simulink model "SimControladorPI"  (R2025b)
settings: Solver=VariableStepAuto  StartTime=0.0  StopTime=tfin  MaxStep=0.01  RelTol=1e-3
values from neighbouring files (symbols this model uses):
  A = max(U)    [AllModels.m]    (also in ConfigurarControl.m = 40; Danier.m; Prueba2.m = 40; PruebaSegundoorden.m)
  den = [tao 1]    [ConfigurarControl.m]    (also in Prueba2.m)
  Kc = 2.5    [ConfigurarControl.m]    (also in Prueba2.m)
  Kc_d = 0.5    [ConfigurarControl.m]    (also in Prueba2.m = 0.2)
  Kc_i = 0.5    [ConfigurarControl.m]    (also in Prueba2.m)
  num = Kp    (= 0.83)    [ConfigurarControl.m]    (also in Prueba2.m)
  t_d = ti_d*0.2    (= 3)    [Prueba2.m]
  tdead = 27.8    [ConfigurarControl.m]    (also in Prueba2.m)
  tesc = 5    [ConfigurarControl.m]    (also in Prueba2.m)
  ti = 10    [ConfigurarControl.m]    (also in Prueba2.m = 20)
libraries: slpidlib x1
settings Model: Creator=b03s217  LastModifiedBy=JF
settings SolverCC: AlgebraicLoopSolver=TrustRegion
settings DebuggingCC: UnconnectedInputMsg=warning  UnconnectedOutputMsg=warning  UnconnectedLineMsg=warning
settings ModelReferenceCC: EnableRefExpFcnMdlSchedulingChecks=on
settings RTWCC: GPUComputeCapability=3.5  DLArmComputeVersion=19.05

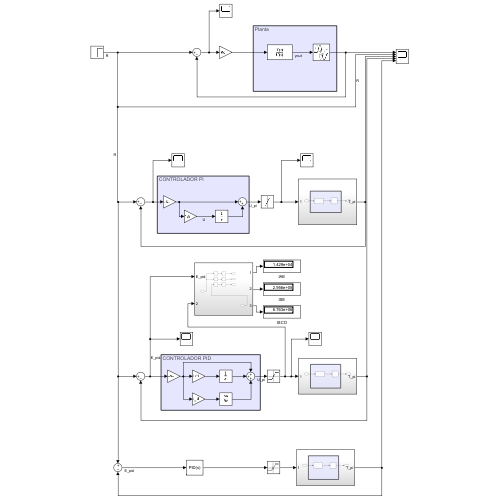
[thumbnail: Simulink's stored preview of the top-level diagram]
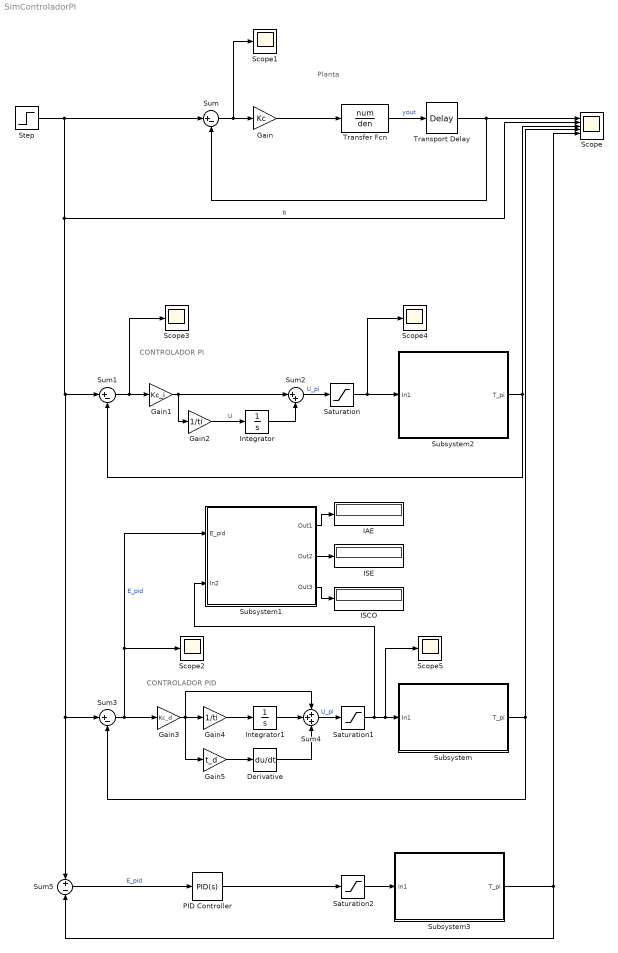
== system SimControladorPI ==
  note: CONTROLADOR PI
  note: CONTROLADOR PID
  note: Planta
  Derivative : Derivative
  Gain : Gain  Gain=Kc
  Gain1 : Gain  Gain=Kc_i
  Gain2 : Gain  Gain=1/ti
  Gain3 : Gain  Gain=Kc_d
  Gain4 : Gain  Gain=1/ti
  Gain5 : Gain  Gain=t_d
  IAE : Display
  ISCO : Display
  ISE : Display
  Integrator : Integrator
  Integrator1 : Integrator
  PID Controller : slpidlib/PID Controller  Controller=PID  Form=Ideal  TimeDomain=Continuous-time  UseExternalTs=off  SampleTime=-1  IntegratorMethod=Forward Euler  FilterMethod=Forward Euler  ControllerParametersSource=internal  P=8.52717951561304  I=0.0130423596873275  UseKiTs=off  D=8.58993288461234  UseExternalDerivativeSource=off  N=3.63365512722758  UseFilter=on  TunerSelectOption=Transfer Function Based (PID Tuner App)  InitialConditionSource=internal  InitialConditionForIntegrator=0  InitialConditionForFilter=0  DifferentiatorICPrevScaledInput=0  ExternalReset=none  TrackingMode=off  Kt=1  LimitOutput=off  SatLimitsSource=internal  UpperSaturationLimit=inf  LowerSaturationLimit=-inf  LinearizeAsGain=on  AntiWindupMode=none  Kb=1  LimitIntegrator=off  UpperIntegratorSaturationLimit=inf  LowerIntegratorSaturationLimit=-inf  POutMin=[]  POutMax=[]  IOutMin=[]  IOutMax=[]  DOutMin=[]  DOutMax=[]  NOutMin=[]  NOutMax=[]  SumOutMin=[]  SumOutMax=[]  SaturationOutMin=[]  SaturationOutMax=[]  PParamMin=[]  PParamMax=[]  IParamMin=[]  IParamMax=[]  DParamMin=[]  DParamMax=[]  NParamMin=[]  NParamMax=[]  KbParamMin=[]  KbParamMax=[]  KtParamMin=[]  KtParamMax=[]  KbOutMin=[]  KbOutMax=[]  KtOutMin=[]  KtOutMax=[]  IntegratorOutMin=[]  IntegratorOutMax=[]  FilterOutMin=[]  FilterOutMax=[]  SumI1OutMin=[]  SumI1OutMax=[]  SumI2OutMin=[]  SumI2OutMax=[]  SumI3OutMin=[]  SumI3OutMax=[]  SumI4OutMin=[]  SumI4OutMax=[]  SumDOutMin=[]  SumDOutMax=[]  DifferentiatorOutMin=[]  DifferentiatorOutMax=[]  FilterDiffOutCoefMin=[]  FilterDiffOutCoefMax=[]  ReciprocalOutMin=[]  ReciprocalOutMax=[]  SumDenOutMin=[]  SumDenOutMax=[]  SumNumOutMin=[]  SumNumOutMax=[]  DivideOutMin=[]  DivideOutMax=[]  UdiffTsProdOutMin=[]  UdiffTsProdOutMax=[]  NTsProdOutMin=[]  NTsProdOutMax=[]  UintegralTsProdOutMin=[]  UintegralTsProdOutMax=[]  UngainTsProdOutMin=[]  UngainTsProdOutMax=[]  ClampingZeroOutDataTypeStr=Inherit: Inherit via back propagation  ClampingZeroOutMin=[]  ClampingZeroOutMax=[]  FilterDenConstantOutDataTypeStr=Inherit: Inherit via back propagation  FilterDenConstantOutMin=[]  FilterDenConstantOutMax=[]  PCopyOutDataTypeStr=Inherit: Inherit via back propagation  PCopyOutMin=[]  PCopyOutMax=[]  NCopyOutDataTypeStr=Inherit: Inherit via back propagation  NCopyOutMin=[]  NCopyOutMax=[]  IntegratorContinuousStateAttributes=''  IntegratorStateMustResolveToSignalObject=off  IntegratorRTWStateStorageClass=Auto  FilterContinuousStateAttributes=''  FilterStateMustResolveToSignalObject=off  FilterRTWStateStorageClass=Auto  ParallelPVariant=Passthrough  IdealPVariant=InternalParameters  IVariant=InternalParameters  DVariant=InternalParameters  IntegratorVariant=Continuous  SatVariant=Disabled  AWVariant=Passthrough  PCopyVariant=Disabled  TRVariant=Disabled  FdbkBlocksVariant=Forward  IdealPFdbkVariant=Disabled  SatFdbkVariant=Disabled  DerivativeFilterVariant=ContFilter  NVariant=InternalParameters  NCopyVariant=Disabled  FilterICVariant=InternalICsFilter  IntegratorICVariant=InternalICs  ExternalResetVariant=Disabled  TRSumVariant=Passthrough  SumFdbkVariant=Disabled  SumVariant=Sum_PID  TsampFilterVariant=InternalTs  TsampNgainVariant=Passthrough  TsampIntegralVariant=Disabled_SignalSpec  ExternalSaturationOutDataTypeStr=Inherit: Same as second input  DerivativeSourceVariant=ErrorSignal  PreIntVariant=InternalPreInt
  Saturation : Saturate  UpperLimit=100  LowerLimit=0
  Saturation1 : Saturate  UpperLimit=100  LowerLimit=0
  Saturation2 : Saturate  UpperLimit=100  LowerLimit=0
  Scope : Scope  NumInputPorts=5
      settings: ActiveDisplayYMinimum=-52.962855985065943  ActiveDisplayYMaximum=83.160796207359652  DataLoggingVariableName=DatosOut
  Scope{1..5} (5 alike) : Scope
      Scope1 settings: ActiveDisplayYMinimum=-4.9999999999999991  ActiveDisplayYMaximum=45
      Scope2 settings: ActiveDisplayYMinimum=-4.9999999999999991  ActiveDisplayYMaximum=45  DataLoggingVariableName=ScopeData2
      Scope3 settings: ActiveDisplayYMinimum=-4.9999999999999991  ActiveDisplayYMaximum=45
      Scope4 settings: ActiveDisplayYMinimum=-4.9999999999999991  ActiveDisplayYMaximum=45  DataLoggingVariableName=ScopeData3
      Scope5 settings: ActiveDisplayYMinimum=-4.9999999999999991  ActiveDisplayYMaximum=45  DataLoggingVariableName=ScopeData4
  Step : Step  Time=tesc  After=A  SampleTime=0
  Subsystem : Subsystem
  Subsystem1 : Subsystem
  Subsystem2 : Subsystem
  Subsystem3 : Subsystem
  Sum : Sum  Inputs=|+-
  Sum1 : Sum  Inputs=|+-
  Sum2 : Sum  Inputs=|++
  Sum3 : Sum  Inputs=|+-
  Sum4 : Sum  Inputs=+++
  Sum5 : Sum  Inputs=+-
  Transfer Fcn : TransferFcn  Numerator=num  Denominator=den
  Transport Delay : TransportDelay  DelayTime=tdead
  wires:
  Transfer Fcn/1 -> Transport Delay/1  "yout"
  Transport Delay/1 -> Sum/2, Scope/1
  Gain/1 -> Transfer Fcn/1
  Sum/1 -> Scope1/1, Gain/1
  Sum1/1 -> Scope3/1, Gain1/1
  Step/1 -> Sum/1, Scope/2, Sum1/1, Sum5/1, Sum3/1  "R"
  Gain2/1 -> Integrator/1  "U"
  Gain1/1 -> Gain2/1, Sum2/1
  Gain4/1 -> Integrator1/1
  Sum3/1 -> Gain3/1, Subsystem1/1(E_pid), Scope2/1  "E_pid"
  Gain3/1 -> Gain5/1, Gain4/1, Sum4/1
  Integrator1/1 -> Sum4/2
  Gain5/1 -> Derivative/1
  Derivative/1 -> Sum4/3
  Sum2/1 -> Saturation/1  "U_pi"
  Saturation/1 -> Scope4/1, Subsystem2/1(In1)
  Sum4/1 -> Saturation1/1  "U_pi"
  Saturation1/1 -> Subsystem1/2(In2), Scope5/1, Subsystem/1(In1)
  Integrator/1 -> Sum2/2
  Subsystem/1(T_pi) -> Scope/4, Sum3/2
  Subsystem1/1(Out1) -> IAE/1
  Subsystem1/2(Out2) -> ISE/1
  Subsystem1/3(Out3) -> ISCO/1
  Subsystem2/1(T_pi) -> Scope/3, Sum1/2
  Saturation2/1 -> Subsystem3/1(In1)
  Sum5/1 -> PID Controller/1  "E_pid"
  PID Controller/1 -> Saturation2/1
  Subsystem3/1(T_pi) -> Scope/5, Sum5/2

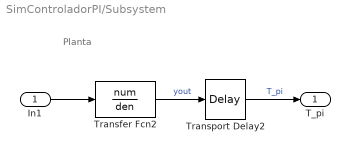
== system SimControladorPI/Subsystem ==
  note: Planta
  In1 : Inport
  Transfer Fcn2 : TransferFcn  Numerator=num  Denominator=den
  Transport Delay2 : TransportDelay  DelayTime=tdead
  T_pi : Outport
  wires:
  Transfer Fcn2/1 -> Transport Delay2/1  "yout"
  Transport Delay2/1 -> T_pi/1  "T_pi"
  In1/1 -> Transfer Fcn2/1

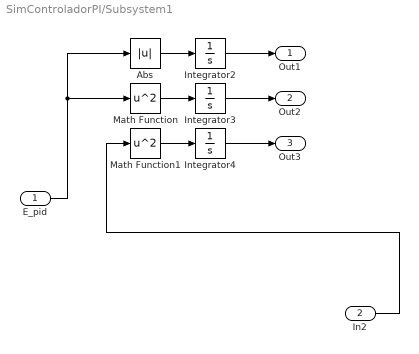
== system SimControladorPI/Subsystem1 ==
  E_pid : Inport
  In2 : Inport  Port=2
  Abs : Abs  SaturateOnIntegerOverflow=off
  Integrator2 : Integrator
  Integrator3 : Integrator
  Integrator4 : Integrator
  Math Function : Math  Operator=square
  Math Function1 : Math  Operator=square
  Out1 : Outport
  Out2 : Outport  Port=2
  Out3 : Outport  Port=3
  wires:
  E_pid/1 -> Math Function/1, Abs/1
  Math Function/1 -> Integrator3/1
  Integrator4/1 -> Out3/1
  Abs/1 -> Integrator2/1
  Math Function1/1 -> Integrator4/1
  Integrator3/1 -> Out2/1
  In2/1 -> Math Function1/1
  Integrator2/1 -> Out1/1

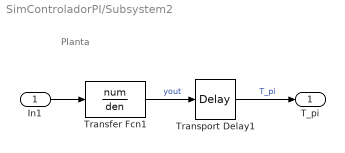
== system SimControladorPI/Subsystem2 ==
  note: Planta
  In1 : Inport
  Transfer Fcn1 : TransferFcn  Numerator=num  Denominator=den
  Transport Delay1 : TransportDelay  DelayTime=tdead
  T_pi : Outport
  wires:
  Transfer Fcn1/1 -> Transport Delay1/1  "yout"
  In1/1 -> Transfer Fcn1/1
  Transport Delay1/1 -> T_pi/1  "T_pi"

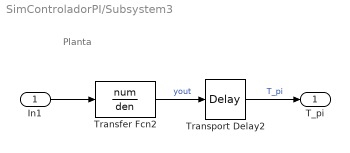
== system SimControladorPI/Subsystem3 ==
  note: Planta
  In1 : Inport
  Transfer Fcn2 : TransferFcn  Numerator=num  Denominator=den
  Transport Delay2 : TransportDelay  DelayTime=tdead
  T_pi : Outport
  wires:
  In1/1 -> Transfer Fcn2/1
  Transport Delay2/1 -> T_pi/1  "T_pi"
  Transfer Fcn2/1 -> Transport Delay2/1  "yout"
